simulink model "singleMassMPCDemo2017"  (R2017a)
settings: Solver=ode4  StartTime=0.0  StopTime=8  FixedStep=0.1  RelTol=1e-3
libraries: simulink x2
settings Model: Creator=daoist  LastModifiedBy=daoist
settings DataIOCC: ReturnWorkspaceOutputs=on
settings DebuggingCC: SFMachineParentedDataDiag=error
settings SFSimCC: SimUseLocalCustomCode=on
settings RTWCC: RTWUseLocalCustomCode=on

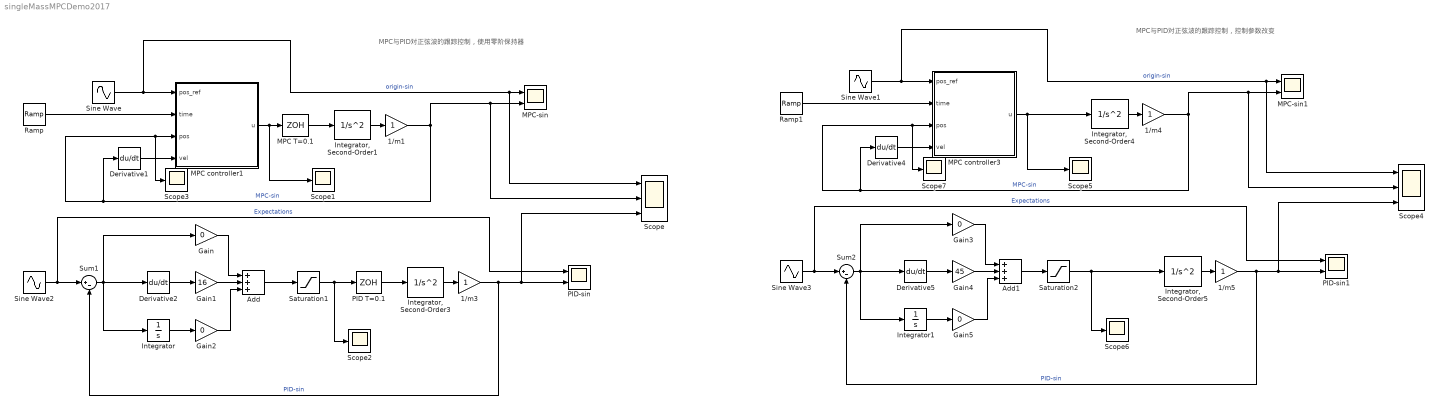
== system singleMassMPCDemo2017 ==
  note: MPC与PID对正弦波的跟踪控制，使用零阶保持器
  note: MPC与PID对正弦波的跟踪控制，控制参数改变
  1/m{1,3..5} (4 alike) : Gain
  Add : Sum  Inputs=+++
  Add1 : Sum  Inputs=+++
  Derivative{1..2,4..5} (4 alike) : Derivative
  Gain{,2..3,5} (4 alike) : Gain  Gain=0
  Gain1 : Gain  Gain=16
  Gain4 : Gain  Gain=45
  Integrator : Integrator
  Integrator, Second-Order{1,3..5} (4 alike) : SecondOrderIntegrator  ShowOutput=x
  Integrator1 : Integrator
  MPC T=0.1 : ZeroOrderHold  SampleTime=0.1
  MPC controller1 : MATLAB Function  TreatAsAtomicUnit=on
  MPC controller3 : MATLAB Function  TreatAsAtomicUnit=on
  MPC-sin : Scope  NumInputPorts=2
  MPC-sin1 : Scope  NumInputPorts=2
  PID T=0.1 : ZeroOrderHold  SampleTime=0.1
  PID-sin : Scope  NumInputPorts=2
  PID-sin1 : Scope  NumInputPorts=2
  Ramp : simulink/Sources/Ramp  slope=1  start=0  X0=0
  Ramp1 : simulink/Sources/Ramp  slope=1  start=0  X0=0
  Saturation1 : Saturate  UpperLimit=100  LowerLimit=-100
  Saturation2 : Saturate  UpperLimit=100  LowerLimit=-100
  Scope : Scope  NumInputPorts=3
  Scope{1..3,5..7} (6 alike) : Scope
  Scope4 : Scope  NumInputPorts=3
  Sine Wave{,1..3} (4 alike) : Sin  Frequency=pi  SampleTime=0
  Sum1 : Sum  Inputs=|+-
  Sum2 : Sum  Inputs=|+-
  wires:
  Derivative1/1 -> MPC controller1/4(vel)
  MPC controller1/1(u) -> Scope1/1, MPC T=0.1/1
  Sine Wave/1 -> Scope/1, MPC-sin/1, MPC controller1/1(pos_ref)  "origin-sin"
  1/m1/1 -> Scope/2, MPC-sin/2, Scope3/1, MPC controller1/3(pos), Derivative1/1  "MPC-sin"
  "Integrator, Second-Order1"/1 -> 1/m1/1
  Ramp/1 -> MPC controller1/2(time)
  1/m3/1 -> Scope/3, PID-sin/2, Sum1/2  "PID-sin"
  Saturation1/1 -> PID T=0.1/1, Scope2/1
  Sine Wave2/1 -> Sum1/1, PID-sin/1  "Expectations"
  "Integrator, Second-Order3"/1 -> 1/m3/1
  Gain1/1 -> Add/2
  Add/1 -> Saturation1/1
  Gain/1 -> Add/1
  Gain2/1 -> Add/3
  Sum1/1 -> Integrator/1, Derivative2/1, Gain/1
  Derivative2/1 -> Gain1/1
  Integrator/1 -> Gain2/1
  PID T=0.1/1 -> "Integrator, Second-Order3"/1
  MPC T=0.1/1 -> "Integrator, Second-Order1"/1
  Derivative5/1 -> Gain4/1
  Sine Wave3/1 -> Sum2/1, PID-sin1/1  "Expectations"
  Integrator1/1 -> Gain5/1
  1/m5/1 -> Scope4/3, PID-sin1/2, Sum2/2  "PID-sin"
  "Integrator, Second-Order5"/1 -> 1/m5/1
  MPC controller3/1(u) -> "Integrator, Second-Order4"/1, Scope5/1
  Sine Wave1/1 -> Scope4/1, MPC-sin1/1, MPC controller3/1(pos_ref)  "origin-sin"
  Ramp1/1 -> MPC controller3/2(time)
  Sum2/1 -> Integrator1/1, Derivative5/1, Gain3/1
  Gain5/1 -> Add1/3
  1/m4/1 -> Scope4/2, MPC-sin1/2, Scope7/1, MPC controller3/3(pos), Derivative4/1  "MPC-sin"
  Gain4/1 -> Add1/2
  Add1/1 -> Saturation2/1
  Derivative4/1 -> MPC controller3/4(vel)
  "Integrator, Second-Order4"/1 -> 1/m4/1
  Gain3/1 -> Add1/1
  Saturation2/1 -> "Integrator, Second-Order5"/1, Scope6/1

== matlab function singleMassMPCDemo2017/MPC controller1 ==
  data: pos_ref input size=1; time input; pos input size=1; vel input size=1; u output size=1
function u = MPCcontroller(pos_ref, time, pos, vel)
%参数设置
m    = 1.05;          %滑块质量,增加了5%作为建模误差
T    = 0.1;           %控制周期100ms
p    = 40;            %控制时域（预测时域）
Q    = 10*eye(2*p);   %累计误差权重
W    = 0.0001*eye(p); %控制输出权重
% umax = 100;          
umax = 100 * ones(p); %控制量限制，即最大的力
Rk   = zeros(2*p,1);  %参考值序列
timeseris = time:T:time+T*(p-1);
Rk(1:2:end) = sin(pi()*(timeseris ))*1.05;    
Rk(2:2:end) = pi()*cos(pi()*(timeseris))*1.05;    %参考速度
%构建中间变量
xk    = [pos;vel];    %xk
A_    = [1 T;0 1];    %离散化预测模型参数A
B_    = [0;T/m];      %离散化预测模型参数B
psi   = zeros(2*p,2); %psi
for i=1:1:p
    psi(i*2-1:i*2,1:2)=A_^i;
end
theta = zeros(2*p,p); %theta
for i=1:1:p
    for j=1:1:i
        theta(i*2-1:i*2,j)=A_^(i-j)*B_;
    end
end
E = psi*xk-Rk;            %E
H = 2*(theta'*Q*theta+W); %H
f = (2*E'*Q*theta)';      %f
%优化求解
coder.extrinsic('quadprog');
Uk=quadprog(H,f,[],[],[],[],-umax,umax);
%返回控制量序列第一个值
u = 0.0;                %显示指定u的类型
u = Uk(1);

== matlab function singleMassMPCDemo2017/MPC controller3 ==
  data: pos_ref input size=1; time input; pos input size=1; vel input size=1; u output size=1
function u = MPCcontroller(pos_ref, time, pos, vel)
%参数设置
m    = 1.05;          %滑块质量,增加了5%作为建模误差
T    = 0.1;           %控制周期100ms
p    = 40;            %控制时域（预测时域）
Q    = 10*eye(2*p);   %累计误差权重
W    = 0.0001*eye(p); %控制输出权重
% umax = 100;          
umax = 100 * ones(p); %控制量限制，即最大的力
Rk   = zeros(2*p,1);  %参考值序列
timeseris = time:T:time+T*(p-1);
Rk(1:2:end) = sin(pi()*(timeseris ))*1.1;    
Rk(2:2:end) = pi()*cos(pi()*(timeseris))*1.1;    %参考速度
%构建中间变量
xk    = [pos;vel];    %xk
A_    = [1 T;0 1];    %离散化预测模型参数A
B_    = [0;T/m];      %离散化预测模型参数B
psi   = zeros(2*p,2); %psi
for i=1:1:p
    psi(i*2-1:i*2,1:2)=A_^i;
end
theta = zeros(2*p,p); %theta
for i=1:1:p
    for j=1:1:i
        theta(i*2-1:i*2,j)=A_^(i-j)*B_;
    end
end
E = psi*xk-Rk;            %E
H = 2*(theta'*Q*theta+W); %H
f = (2*E'*Q*theta)';      %f
%优化求解
coder.extrinsic('quadprog');
Uk=quadprog(H,f,[],[],[],[],-umax,umax);
%返回控制量序列第一个值
u = 0.0;                %显示指定u的类型
u = Uk(1);
